simulink model "Nexonar_Navigation1"  (R2018b)
settings: Solver=FixedStepDiscrete  StartTime=0.0  StopTime=0.1  RelTol=1e-3  EnableMultiTasking=on
libraries: commutil2 x12, c280xlib x3, c2833xlib x2, c2000lib x1
settings Model: ExtModeTrigDuration=8  Creator=User  LastModifiedBy=hengw
settings DataIOCC: LimitDataPoints=on  SaveFormat=Array  SaveOutput=off  SaveTime=off
settings OptimizationCC: DefaultUnderspecifiedDataType=single  ExpressionDepthLimit=2147483647  LifeSpan=1  MaxStackSize=512
settings DebuggingCC: UnderspecifiedInitializationDetection=Classic  MergeDetectMultiDrivingBlocksExec=none  SolverPrmCheckMsg=warning  StateNameClashWarn=warning  SFUnexpectedBacktrackingDiag=warning  SFNoUnconditionalDefaultTransitionDiag=warning  SFExecutionAtInitializationDiag=none
settings HardwareCC: ProdBitPerChar=16  ProdBitPerInt=16  ProdBitPerPointer=32  ProdBitPerSizeT=32  ProdBitPerPtrDiffT=32  ProdLargestAtomicInteger=Integer  ProdLargestAtomicFloat=None  ProdWordSize=16  ProdLongLongMode=on  ProdHWDeviceType=Texas Instruments->C2000  TargetBitPerChar=16  TargetBitPerInt=16  TargetLargestAtomicInteger=Integer  TargetIntDivRoundTo=Zero  TargetEndianess=LittleEndian  TargetWordSize=16  TargetHWDeviceType=Texas Instruments->C2000  ProdEqTarget=off
settings ModelReferenceCC: PropagateSignalLabelsOutOfModel=off
settings SFSimCC: SimCustomSourceCode="#include \"i2c_reset.c\""  SimCustomHeaderCode="#include \"i2c_reset.h\""  SimUseLocalCustomCode=off  MATLABDynamicMemAlloc=off
settings RTWCC: SystemTargetFile=ert.tlc  HardwareBoard=TI Delfino F2833x  TemplateMakefile=ert_default_tmf  RTWUseLocalCustomCode=off  RTWUseSimCustomCode=on  CustomSourceCode="#include \"i2c_reset.c\""  CustomHeaderCode="#include \"i2c_reset.h\""  Toolchain=Texas Instruments Code Composer Studio (C2000)
settings CodeAppCC: IgnoreCustomStorageClasses=off  CustomSymbolStrType=$N$R$M  StateflowObjectComments=on  InternalIdentifier=Classic
settings ERTTargetCC: CodeReplacementLibrary=TI C28x  MultiwordLength=2048  ParMdlRefBuildCompliant=off  CPPClassGenCompliant=off  ConvertIfToSwitch=off  SuppressUnreachableDefaultCases=off
settings ConfigComp: CovMetricSettings=dw  CovHtmlReporting=on  CovSaveCumulativeToWorkspaceVar=on  CovSaveSingleToWorkspaceVar=on  CovExternalEMLEnable=off  PSAutoStubLUT=on

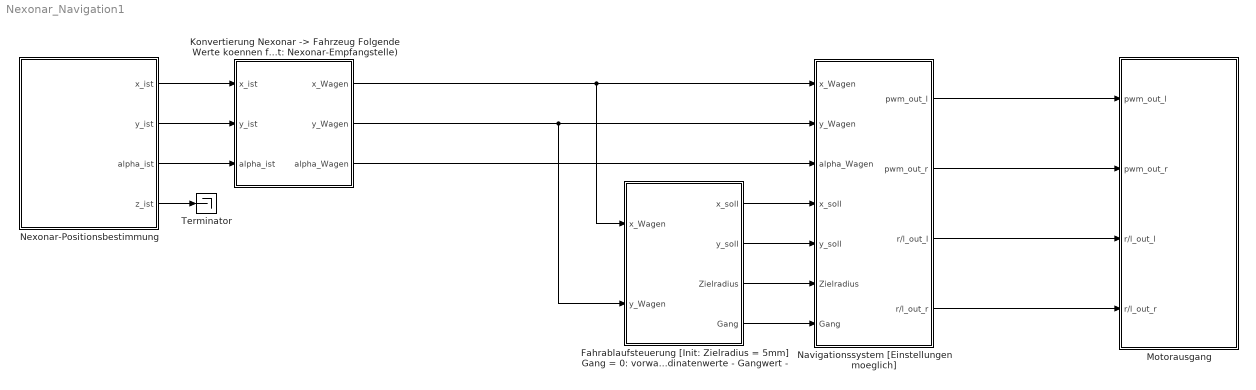
== system Nexonar_Navigation1 ==
  "Fahrablaufsteuerung [Init: Zielradius = 5mm] Gang = 0: vorwaerts Gang = 1: rueckwaerts Folgende Werte fuer den Ablauf sind einstellbar: - Zielkoordinatenwerte - Gangwert - " : Stateflow chart  TreatAsAtomicUnit=on
  "Konvertierung Nexonar -> Fahrzeug Folgende Werte koennen für Nexonar eingestellt werden: - r_Versatz_Nexo: Radialer Versatz des Nexonars zur Rotationsachse des Fahrzeugs - phi_Versatz_Nexo: Winkelversatz des Nexonars gegenüber der x-Achse (Mittelpunkt: Rotationspunkt des Fahrzeugs) - psi_Offset_Nexo: Winkelversatz des Nexonars gegenüber der x-Achse (Mittelpunkt: Nexonar-Empfangstelle)" : MATLAB Function  TreatAsAtomicUnit=on
  Motorausgang : Subsystem
  Navigationssystem [Einstellungen moeglich] : Subsystem  TreatAsAtomicUnit=on
  Nexonar-Positionsbestimmung : Subsystem
  Terminator : Terminator
  wires:
  Navigationssystem [Einstellungen moeglich]/2(pwm_out_r) -> Motorausgang/2(pwm_out_r)
  "Fahrablaufsteuerung [Init: Zielradius = 5mm] Gang = 0: vorwaerts Gang = 1: rueckwaerts Folgende Werte fuer den Ablauf sind einstellbar: - Zielkoordinatenwerte - Gangwert - "/2(y_soll) -> Navigationssystem [Einstellungen moeglich]/5(y_soll)
  Navigationssystem [Einstellungen moeglich]/3(r/l_out_l) -> Motorausgang/3(r/l_out_l)
  "Fahrablaufsteuerung [Init: Zielradius = 5mm] Gang = 0: vorwaerts Gang = 1: rueckwaerts Folgende Werte fuer den Ablauf sind einstellbar: - Zielkoordinatenwerte - Gangwert - "/4(Gang) -> Navigationssystem [Einstellungen moeglich]/7(Gang)
  "Fahrablaufsteuerung [Init: Zielradius = 5mm] Gang = 0: vorwaerts Gang = 1: rueckwaerts Folgende Werte fuer den Ablauf sind einstellbar: - Zielkoordinatenwerte - Gangwert - "/1(x_soll) -> Navigationssystem [Einstellungen moeglich]/4(x_soll)
  "Fahrablaufsteuerung [Init: Zielradius = 5mm] Gang = 0: vorwaerts Gang = 1: rueckwaerts Folgende Werte fuer den Ablauf sind einstellbar: - Zielkoordinatenwerte - Gangwert - "/3(Zielradius) -> Navigationssystem [Einstellungen moeglich]/6(Zielradius)
  "Konvertierung Nexonar -> Fahrzeug Folgende Werte koennen für Nexonar eingestellt werden: - r_Versatz_Nexo: Radialer Versatz des Nexonars zur Rotationsachse des Fahrzeugs - phi_Versatz_Nexo: Winkelversatz des Nexonars gegenüber der x-Achse (Mittelpunkt: Rotationspunkt des Fahrzeugs) - psi_Offset_Nexo: Winkelversatz des Nexonars gegenüber der x-Achse (Mittelpunkt: Nexonar-Empfangstelle)"/2(y_Wagen) -> "Fahrablaufsteuerung [Init: Zielradius = 5mm] Gang = 0: vorwaerts Gang = 1: rueckwaerts Folgende Werte fuer den Ablauf sind einstellbar: - Zielkoordinatenwerte - Gangwert - "/2(y_Wagen), Navigationssystem [Einstellungen moeglich]/2(y_Wagen)
  Navigationssystem [Einstellungen moeglich]/4(r/l_out_r) -> Motorausgang/4(r/l_out_r)
  "Konvertierung Nexonar -> Fahrzeug Folgende Werte koennen für Nexonar eingestellt werden: - r_Versatz_Nexo: Radialer Versatz des Nexonars zur Rotationsachse des Fahrzeugs - phi_Versatz_Nexo: Winkelversatz des Nexonars gegenüber der x-Achse (Mittelpunkt: Rotationspunkt des Fahrzeugs) - psi_Offset_Nexo: Winkelversatz des Nexonars gegenüber der x-Achse (Mittelpunkt: Nexonar-Empfangstelle)"/1(x_Wagen) -> "Fahrablaufsteuerung [Init: Zielradius = 5mm] Gang = 0: vorwaerts Gang = 1: rueckwaerts Folgende Werte fuer den Ablauf sind einstellbar: - Zielkoordinatenwerte - Gangwert - "/1(x_Wagen), Navigationssystem [Einstellungen moeglich]/1(x_Wagen)
  Navigationssystem [Einstellungen moeglich]/1(pwm_out_l) -> Motorausgang/1(pwm_out_l)
  Nexonar-Positionsbestimmung/4(z_ist) -> Terminator/1
  "Konvertierung Nexonar -> Fahrzeug Folgende Werte koennen für Nexonar eingestellt werden: - r_Versatz_Nexo: Radialer Versatz des Nexonars zur Rotationsachse des Fahrzeugs - phi_Versatz_Nexo: Winkelversatz des Nexonars gegenüber der x-Achse (Mittelpunkt: Rotationspunkt des Fahrzeugs) - psi_Offset_Nexo: Winkelversatz des Nexonars gegenüber der x-Achse (Mittelpunkt: Nexonar-Empfangstelle)"/3(alpha_Wagen) -> Navigationssystem [Einstellungen moeglich]/3(alpha_Wagen)
  Nexonar-Positionsbestimmung/1(x_ist) -> "Konvertierung Nexonar -> Fahrzeug Folgende Werte koennen für Nexonar eingestellt werden: - r_Versatz_Nexo: Radialer Versatz des Nexonars zur Rotationsachse des Fahrzeugs - phi_Versatz_Nexo: Winkelversatz des Nexonars gegenüber der x-Achse (Mittelpunkt: Rotationspunkt des Fahrzeugs) - psi_Offset_Nexo: Winkelversatz des Nexonars gegenüber der x-Achse (Mittelpunkt: Nexonar-Empfangstelle)"/1(x_ist)
  Nexonar-Positionsbestimmung/2(y_ist) -> "Konvertierung Nexonar -> Fahrzeug Folgende Werte koennen für Nexonar eingestellt werden: - r_Versatz_Nexo: Radialer Versatz des Nexonars zur Rotationsachse des Fahrzeugs - phi_Versatz_Nexo: Winkelversatz des Nexonars gegenüber der x-Achse (Mittelpunkt: Rotationspunkt des Fahrzeugs) - psi_Offset_Nexo: Winkelversatz des Nexonars gegenüber der x-Achse (Mittelpunkt: Nexonar-Empfangstelle)"/2(y_ist)
  Nexonar-Positionsbestimmung/3(alpha_ist) -> "Konvertierung Nexonar -> Fahrzeug Folgende Werte koennen für Nexonar eingestellt werden: - r_Versatz_Nexo: Radialer Versatz des Nexonars zur Rotationsachse des Fahrzeugs - phi_Versatz_Nexo: Winkelversatz des Nexonars gegenüber der x-Achse (Mittelpunkt: Rotationspunkt des Fahrzeugs) - psi_Offset_Nexo: Winkelversatz des Nexonars gegenüber der x-Achse (Mittelpunkt: Nexonar-Empfangstelle)"/3(alpha_ist)

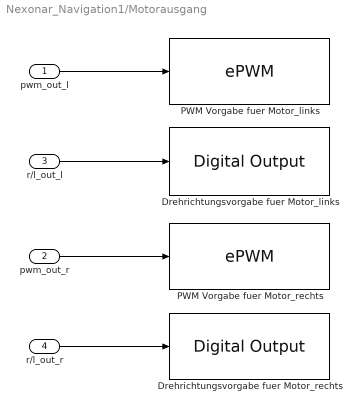
== system Nexonar_Navigation1/Motorausgang ==
  pwm_out_l : Inport
  pwm_out_r : Inport  Port=2
  r/l_out_l : Inport  Port=3
  r/l_out_r : Inport  Port=4
  Drehrichtungsvorgabe fuer Motor_links : c2833xlib/Digital Output  GPIO_Number=GPIO16~GPIO23  GPIO_Bit0=off  GPIO_BIT0_Toggle=off  GPIO_Bit1=off  GPIO_BIT1_Toggle=off  GPIO_Bit2=off  GPIO_BIT2_Toggle=off  GPIO_Bit3=off  GPIO_BIT3_Toggle=off  GPIO_Bit4=on  GPIO_BIT4_Toggle=off  GPIO_Bit5=off  GPIO_BIT5_Toggle=off  GPIO_Bit6=off  GPIO_BIT6_Toggle=off  GPIO_Bit7=off  GPIO_BIT7_Toggle=off
      settings: SourceProductName=Embedded Coder Support Package for Texas Instruments C2000 Processors  SourceProductBaseCode=TIC2000
  Drehrichtungsvorgabe fuer Motor_rechts : c2833xlib/Digital Output  GPIO_Number=GPIO16~GPIO23  GPIO_Bit0=off  GPIO_BIT0_Toggle=off  GPIO_Bit1=off  GPIO_BIT1_Toggle=off  GPIO_Bit2=off  GPIO_BIT2_Toggle=off  GPIO_Bit3=off  GPIO_BIT3_Toggle=off  GPIO_Bit4=off  GPIO_BIT4_Toggle=off  GPIO_Bit5=on  GPIO_BIT5_Toggle=off  GPIO_Bit6=off  GPIO_BIT6_Toggle=off  GPIO_Bit7=off  GPIO_BIT7_Toggle=off
      settings: SourceProductName=Embedded Coder Support Package for Texas Instruments C2000 Processors  SourceProductBaseCode=TIC2000
  "PWM Vorgabe fuer Motor_links " : c280xlib/ePWM  checkMode=off  useModule=ePWM1  periodUnits=Clock cycles  timerSource=Specify via dialog  timerPeriod_clk=64000  timerPeriod_sec=0.0001  tbshadow=Counter equals to zero  countingMode=Up  phaseActiveEnable=Disable  phaseDirection=Count down after sync  phaseActive=0  synchronizationEnable=off  synchronizationOption=Disable  clockPrescale=1  HSclockPrescale=1  ePWMxAStatus=off  CMPAUnits=Clock cycles  CMPASource=Specify via dialog  CMPAValue_per=50  CMPAValue_clk=32000  enCMPAshadow=Counter equals to zero  ePWMxAactionLogic1=Do nothing  ePWMxAactionLogic2=Clear  ePWMxAactionLogic3=Set  ePWMxAactionLogic4=Do nothing  ePWMxAactionLogic5=Do nothing  ePWMxAactionLogic6=Do nothing  ePWMxALoadMode=Load on counter equals to zero (CTR=Zero)  ePWMxACSFenable=off  ePWMxACSFvalue=Forcing disable  ePWMxASFreload=Zero  enHRPWM=off  HRPWM_LoadMode=Counter equals to zero (CTR=ZERO)  HRPWM_CTLMode=Phase control mode  HRPWM_EDGMode=Both edge  enSFO=on  ePWMxBStatus=on  CMPBUnits=Percentages  CMPBSource=Input port  CMPBValue_per=0  CMPBValue_clk=32000  enCMPBshadow=Counter equals to zero  ePWMxBactionLogic1=Do nothing  ePWMxBactionLogic2=Set  ePWMxBactionLogic3=Do nothing  ePWMxBactionLogic4=Do nothing  ePWMxBactionLogic5=Clear  ePWMxBactionLogic6=Do nothing  ePWMxBLoadMode=Load on counter equals to zero (CTR=Zero)  ePWMxBCSFenable=off  ePWMxBCSFvalue=Forcing disable  ePWMxBSFreload=Zero  enableDBePWMxA=off  enableDBePWMxB=off  DBpolarity=Active high (AH)  DBedgeDelay=Positive  DBSource_ePWMxA=ePWMxA  DBSource_ePWMxB=ePWMxA  DBperiodSource=Specify via dialog  REDperiod=0  FEDperiod=0  adcstartModuleA=off  adcrequestEventA=First event  adcstartEventA=Counter equals to zero (CTR=Zero)  adcstartModuleB=off  adcrequestEventB=First event  adcstartEventB=Counter equals to zero (CTR=Zero)  intEn=off  intPrd=First event  intSel=Counter equals to zero (CTR=Zero)  chopperEnable=off  chopperFrequency=1  chopperFirstwidth=1  chopperDuty=12.5%  tripZonesource=Specify via dialog  tzselOSHT1=off  tzselOSHT2=off  tzselOSHT3=off  tzselOSHT4=off  tzselOSHT5=off  tzselOSHT6=off  tzselCBC1=off  tzselCBC2=off  tzselCBC3=off  tzselCBC4=off  tzselCBC5=off  tzselCBC6=off  enTzOstIntr=off  enTzCbcIntr=off  ePWMxAforced=No action  ePWMxBforced=No action  timerPeriod=-1  ePWMxAValue=0  ePWMxBValue=0  tripZoneoption=One-shot trip (OSHT)
      settings: SourceProductName=Embedded Coder Support Package for Texas Instruments C2000 Processors  SourceProductBaseCode=TIC2000
  PWM Vorgabe fuer Motor_rechts : c280xlib/ePWM  checkMode=off  useModule=ePWM2  periodUnits=Clock cycles  timerSource=Specify via dialog  timerPeriod_clk=64000  timerPeriod_sec=0.0001  tbshadow=Counter equals to zero  countingMode=Up  phaseActiveEnable=Disable  phaseDirection=Count down after sync  phaseActive=0  synchronizationEnable=off  synchronizationOption=Disable  clockPrescale=1  HSclockPrescale=1  ePWMxAStatus=off  CMPAUnits=Clock cycles  CMPASource=Specify via dialog  CMPAValue_per=50  CMPAValue_clk=32000  enCMPAshadow=Counter equals to zero  ePWMxAactionLogic1=Do nothing  ePWMxAactionLogic2=Clear  ePWMxAactionLogic3=Set  ePWMxAactionLogic4=Do nothing  ePWMxAactionLogic5=Do nothing  ePWMxAactionLogic6=Do nothing  ePWMxALoadMode=Load on counter equals to zero (CTR=Zero)  ePWMxACSFenable=off  ePWMxACSFvalue=Forcing disable  ePWMxASFreload=Zero  enHRPWM=off  HRPWM_LoadMode=Counter equals to zero (CTR=ZERO)  HRPWM_CTLMode=Phase control mode  HRPWM_EDGMode=Both edge  enSFO=on  ePWMxBStatus=on  CMPBUnits=Percentages  CMPBSource=Input port  CMPBValue_per=0  CMPBValue_clk=32000  enCMPBshadow=Counter equals to zero  ePWMxBactionLogic1=Do nothing  ePWMxBactionLogic2=Set  ePWMxBactionLogic3=Do nothing  ePWMxBactionLogic4=Do nothing  ePWMxBactionLogic5=Clear  ePWMxBactionLogic6=Do nothing  ePWMxBLoadMode=Load on counter equals to zero (CTR=Zero)  ePWMxBCSFenable=off  ePWMxBCSFvalue=Forcing disable  ePWMxBSFreload=Zero  enableDBePWMxA=off  enableDBePWMxB=off  DBpolarity=Active high (AH)  DBedgeDelay=Positive  DBSource_ePWMxA=ePWMxA  DBSource_ePWMxB=ePWMxA  DBperiodSource=Specify via dialog  REDperiod=0  FEDperiod=0  adcstartModuleA=off  adcrequestEventA=First event  adcstartEventA=Counter equals to zero (CTR=Zero)  adcstartModuleB=off  adcrequestEventB=First event  adcstartEventB=Counter equals to zero (CTR=Zero)  intEn=off  intPrd=First event  intSel=Counter equals to zero (CTR=Zero)  chopperEnable=off  chopperFrequency=1  chopperFirstwidth=1  chopperDuty=12.5%  tripZonesource=Specify via dialog  tzselOSHT1=off  tzselOSHT2=off  tzselOSHT3=off  tzselOSHT4=off  tzselOSHT5=off  tzselOSHT6=off  tzselCBC1=off  tzselCBC2=off  tzselCBC3=off  tzselCBC4=off  tzselCBC5=off  tzselCBC6=off  enTzOstIntr=off  enTzCbcIntr=off  ePWMxAforced=No action  ePWMxBforced=No action  timerPeriod=-1  ePWMxAValue=0  ePWMxBValue=0  tripZoneoption=One-shot trip (OSHT)
      settings: SourceProductName=Embedded Coder Support Package for Texas Instruments C2000 Processors  SourceProductBaseCode=TIC2000
  wires:
  pwm_out_l/1 -> "PWM Vorgabe fuer Motor_links "/1
  pwm_out_r/1 -> PWM Vorgabe fuer Motor_rechts/1
  r/l_out_l/1 -> Drehrichtungsvorgabe fuer Motor_links/1
  r/l_out_r/1 -> Drehrichtungsvorgabe fuer Motor_rechts/1

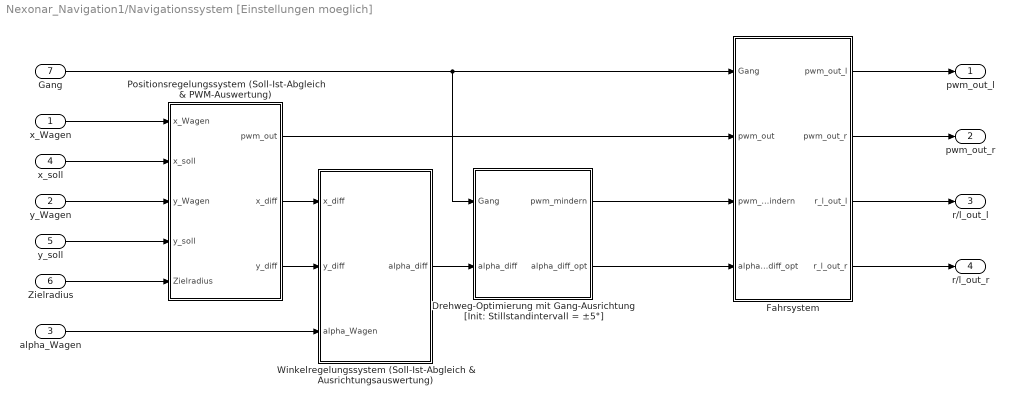
== system Nexonar_Navigation1/Navigationssystem [Einstellungen moeglich] ==
  x_Wagen : Inport
  y_Wagen : Inport  Port=2
  alpha_Wagen : Inport  Port=3
  x_soll : Inport  Port=4
  y_soll : Inport  Port=5
  Zielradius : Inport  Port=6
  Gang : Inport  Port=7
  Drehweg-Optimierung mit Gang-Ausrichtung [Init: Stillstandintervall = ±5°] : Stateflow chart  TreatAsAtomicUnit=on
  Fahrsystem : Stateflow chart  TreatAsAtomicUnit=on
  Positionsregelungssystem (Soll-Ist-Abgleich & PWM-Auswertung) : Subsystem
  Winkelregelungssystem (Soll-Ist-Abgleich & Ausrichtungsauswertung) : Subsystem
  pwm_out_l : Outport
  pwm_out_r : Outport  Port=2
  r/l_out_l : Outport  Port=3
  r/l_out_r : Outport  Port=4
  wires:
  Positionsregelungssystem (Soll-Ist-Abgleich & PWM-Auswertung)/2(x_diff) -> Winkelregelungssystem (Soll-Ist-Abgleich & Ausrichtungsauswertung)/1(x_diff)
  y_soll/1 -> Positionsregelungssystem (Soll-Ist-Abgleich & PWM-Auswertung)/4(y_soll)
  y_Wagen/1 -> Positionsregelungssystem (Soll-Ist-Abgleich & PWM-Auswertung)/3(y_Wagen)
  Gang/1 -> Fahrsystem/1(Gang), Drehweg-Optimierung mit Gang-Ausrichtung [Init: Stillstandintervall = ±5°]/1(Gang)
  Positionsregelungssystem (Soll-Ist-Abgleich & PWM-Auswertung)/3(y_diff) -> Winkelregelungssystem (Soll-Ist-Abgleich & Ausrichtungsauswertung)/2(y_diff)
  x_Wagen/1 -> Positionsregelungssystem (Soll-Ist-Abgleich & PWM-Auswertung)/1(x_Wagen)
  x_soll/1 -> Positionsregelungssystem (Soll-Ist-Abgleich & PWM-Auswertung)/2(x_soll)
  alpha_Wagen/1 -> Winkelregelungssystem (Soll-Ist-Abgleich & Ausrichtungsauswertung)/3(alpha_Wagen)
  Fahrsystem/2(pwm_out_r) -> pwm_out_r/1
  Fahrsystem/4(r_l_out_r) -> r/l_out_r/1
  Fahrsystem/1(pwm_out_l) -> pwm_out_l/1
  Fahrsystem/3(r_l_out_l) -> r/l_out_l/1
  Winkelregelungssystem (Soll-Ist-Abgleich & Ausrichtungsauswertung)/1(alpha_diff) -> Drehweg-Optimierung mit Gang-Ausrichtung [Init: Stillstandintervall = ±5°]/2(alpha_diff)
  Drehweg-Optimierung mit Gang-Ausrichtung [Init: Stillstandintervall = ±5°]/2(alpha_diff_opt) -> Fahrsystem/4(alpha_diff_opt)
  Zielradius/1 -> Positionsregelungssystem (Soll-Ist-Abgleich & PWM-Auswertung)/5(Zielradius)
  Drehweg-Optimierung mit Gang-Ausrichtung [Init: Stillstandintervall = ±5°]/1(pwm_mindern) -> Fahrsystem/3(pwm_mindern)
  Positionsregelungssystem (Soll-Ist-Abgleich & PWM-Auswertung)/1(pwm_out) -> Fahrsystem/2(pwm_out)

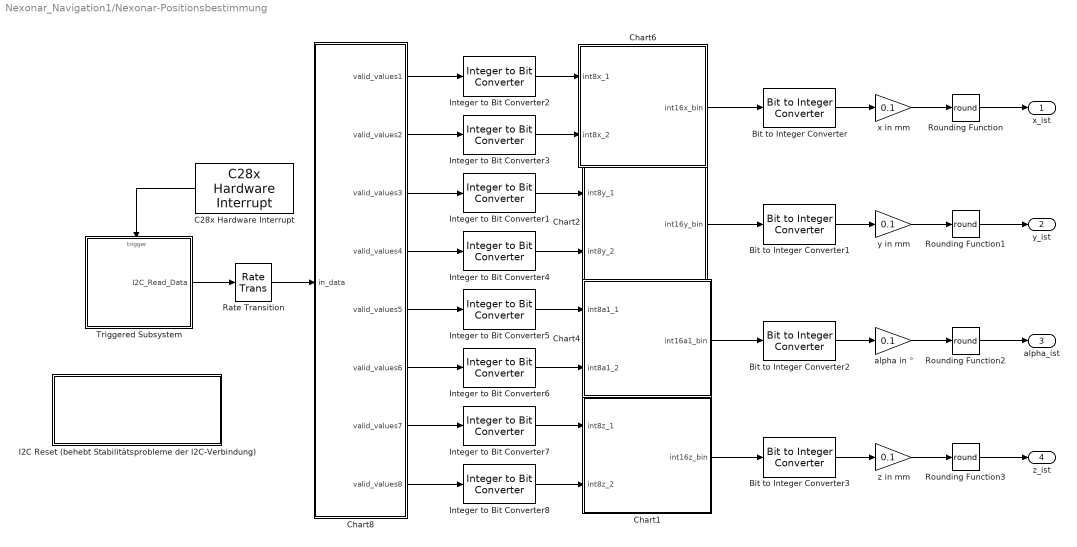
== system Nexonar_Navigation1/Nexonar-Positionsbestimmung ==
  Bit to Integer Converter{,1..3} (4 alike) : commutil2/Bit to Integer Converter  nbits=16  bitOrder=MSB first  signedOutputValues=Signed  outDtype=Inherit via internal rule  outDtypeSigned=Inherit via internal rule
      settings: SourceProductName=Communications Toolbox
  C28x Hardware Interrupt : c2000lib/Scheduling/C28x Hardware Interrupt  irqnumbers=8  pienumbers=2  irqpriorities=30  irqpreempts=0  showinput=off  dspchiptype=C280X
      settings: SourceProductName=Embedded Coder Support Package for Texas Instruments C2000 Processors  SourceProductBaseCode=TIC2000
  Chart1 : Stateflow chart  TreatAsAtomicUnit=on
  Chart2 : Stateflow chart  TreatAsAtomicUnit=on
  Chart4 : Stateflow chart  TreatAsAtomicUnit=on
  Chart6 : Stateflow chart  TreatAsAtomicUnit=on
  Chart8 : Stateflow chart  TreatAsAtomicUnit=on
  I2C Reset (behebt Stabilitätsprobleme der I2C-Verbindung) : Subsystem
  Integer to Bit Converter{1..8} (8 alike) : commutil2/Integer to Bit Converter  nbits=8  signedInputValues=Unsigned  bitOrder=MSB first  outDtype=uint8
      settings: SourceProductName=Communications Toolbox
  Rate Transition : RateTransition  Deterministic=off  OutPortSampleTime=0.01
  Rounding Function{,1..3} (4 alike) : Rounding  Operator=round
  Triggered Subsystem : Subsystem  TreatAsAtomicUnit=on
  alpha in ° : Gain  Gain=0.1  OutDataTypeStr=double
  x in mm : Gain  Gain=0.1  OutDataTypeStr=double
  y in mm : Gain  Gain=0.1  OutDataTypeStr=double
  z in mm : Gain  Gain=0.1  OutDataTypeStr=double
  x_ist : Outport
  y_ist : Outport  Port=2
  alpha_ist : Outport  Port=3
  z_ist : Outport  Port=4
  wires:
  Integer to Bit Converter7/1 -> Chart1/1(int8z_1)
  Integer to Bit Converter8/1 -> Chart1/2(int8z_2)
  Chart8/7(valid_values7) -> Integer to Bit Converter7/1
  Chart8/8(valid_values8) -> Integer to Bit Converter8/1
  Triggered Subsystem/1(I2C_Read_Data) -> Rate Transition/1
  Chart1/1(int16z_bin) -> Bit to Integer Converter3/1
  Chart4/1(int16a1_bin) -> Bit to Integer Converter2/1
  Chart8/6(valid_values6) -> Integer to Bit Converter6/1
  Integer to Bit Converter6/1 -> Chart4/2(int8a1_2)
  Integer to Bit Converter5/1 -> Chart4/1(int8a1_1)
  Integer to Bit Converter4/1 -> Chart2/2(int8y_2)
  Integer to Bit Converter2/1 -> Chart6/1(int8x_1)
  Integer to Bit Converter1/1 -> Chart2/1(int8y_1)
  Chart6/1(int16x_bin) -> Bit to Integer Converter/1
  Integer to Bit Converter3/1 -> Chart6/2(int8x_2)
  Chart8/3(valid_values3) -> Integer to Bit Converter1/1
  Chart8/1(valid_values1) -> Integer to Bit Converter2/1
  Chart2/1(int16y_bin) -> Bit to Integer Converter1/1
  Chart8/4(valid_values4) -> Integer to Bit Converter4/1
  Chart8/2(valid_values2) -> Integer to Bit Converter3/1
  Chart8/5(valid_values5) -> Integer to Bit Converter5/1
  C28x Hardware Interrupt/1 -> Triggered Subsystem/Trigger
  Rate Transition/1 -> Chart8/1(in_data)
  x in mm/1 -> Rounding Function/1
  Bit to Integer Converter/1 -> x in mm/1
  Bit to Integer Converter1/1 -> y in mm/1
  y in mm/1 -> Rounding Function1/1
  Bit to Integer Converter3/1 -> z in mm/1
  z in mm/1 -> Rounding Function3/1
  Bit to Integer Converter2/1 -> alpha in °/1
  alpha in °/1 -> Rounding Function2/1
  Rounding Function/1 -> x_ist/1
  Rounding Function2/1 -> alpha_ist/1
  Rounding Function1/1 -> y_ist/1
  Rounding Function3/1 -> z_ist/1

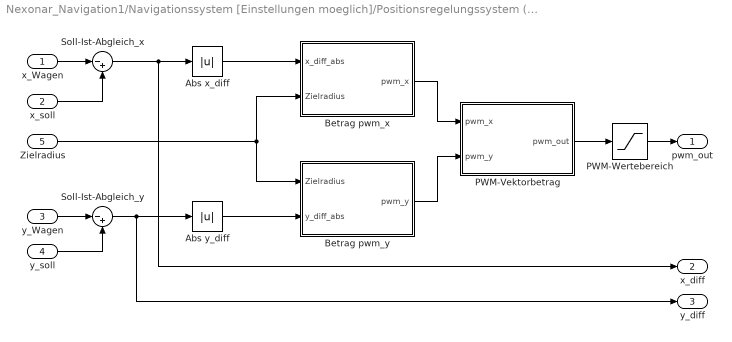
== system Nexonar_Navigation1/Navigationssystem [Einstellungen moeglich]/Positionsregelungssystem (Soll-Ist-Abgleich & PWM-Auswertung) ==
  x_Wagen : Inport
  x_soll : Inport  Port=2
  y_Wagen : Inport  Port=3
  y_soll : Inport  Port=4
  Zielradius : Inport  Port=5
  Abs x_diff : Abs  SampleTime=0.01
  Abs y_diff : Abs  SampleTime=0.01
  Betrag pwm_x : MATLAB Function  TreatAsAtomicUnit=on  SystemSampleTime=0.01
  Betrag pwm_y : MATLAB Function  TreatAsAtomicUnit=on  SystemSampleTime=0.01
  PWM-Vektorbetrag : MATLAB Function  TreatAsAtomicUnit=on
  PWM-Wertebereich : Saturate  UpperLimit=100  LowerLimit=0
  Soll-Ist-Abgleich_x : Sum  Inputs=|-+  SampleTime=0.01
  Soll-Ist-Abgleich_y : Sum  Inputs=|-+  AccumDataTypeStr=double  SampleTime=0.01
  pwm_out : Outport
  x_diff : Outport  Port=2
  y_diff : Outport  Port=3
  wires:
  Soll-Ist-Abgleich_x/1 -> x_diff/1, Abs x_diff/1
  Abs x_diff/1 -> Betrag pwm_x/1(x_diff_abs)
  x_soll/1 -> Soll-Ist-Abgleich_x/2
  x_Wagen/1 -> Soll-Ist-Abgleich_x/1
  y_Wagen/1 -> Soll-Ist-Abgleich_y/1
  y_soll/1 -> Soll-Ist-Abgleich_y/2
  Soll-Ist-Abgleich_y/1 -> Abs y_diff/1, y_diff/1
  Abs y_diff/1 -> Betrag pwm_y/2(y_diff_abs)
  PWM-Wertebereich/1 -> pwm_out/1
  PWM-Vektorbetrag/1(pwm_out) -> PWM-Wertebereich/1
  Betrag pwm_x/1(pwm_x) -> PWM-Vektorbetrag/1(pwm_x)
  Betrag pwm_y/1(pwm_y) -> PWM-Vektorbetrag/2(pwm_y)
  Zielradius/1 -> Betrag pwm_y/1(Zielradius), Betrag pwm_x/2(Zielradius)

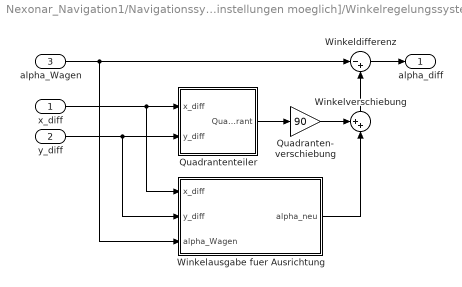
== system Nexonar_Navigation1/Navigationssystem [Einstellungen moeglich]/Winkelregelungssystem (Soll-Ist-Abgleich & Ausrichtungsauswertung) ==
  x_diff : Inport
  y_diff : Inport  Port=2
  alpha_Wagen : Inport  Port=3
  Quadranten- verschiebung : Gain  Gain=90
  Quadrantenteiler : Stateflow chart  TreatAsAtomicUnit=on
  Winkelausgabe fuer Ausrichtung : Stateflow chart  TreatAsAtomicUnit=on
  Winkeldifferenz : Sum  Inputs=|-+
  Winkelverschiebung : Sum  Inputs=++|
  alpha_diff : Outport
  wires:
  alpha_Wagen/1 -> Winkelausgabe fuer Ausrichtung/3(alpha_Wagen), Winkeldifferenz/1
  y_diff/1 -> Winkelausgabe fuer Ausrichtung/2(y_diff), Quadrantenteiler/2(y_diff)
  Winkelausgabe fuer Ausrichtung/1(alpha_neu) -> Winkelverschiebung/2
  Winkelverschiebung/1 -> Winkeldifferenz/2
  x_diff/1 -> Winkelausgabe fuer Ausrichtung/1(x_diff), Quadrantenteiler/1(x_diff)
  Quadrantenteiler/1(Quadrant) -> Quadranten- verschiebung/1
  Winkeldifferenz/1 -> alpha_diff/1
  Quadranten- verschiebung/1 -> Winkelverschiebung/1

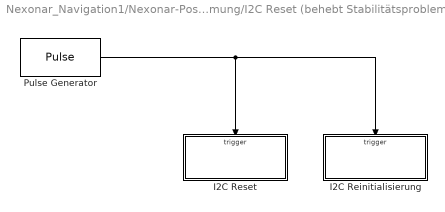
== system Nexonar_Navigation1/Nexonar-Positionsbestimmung/I2C Reset (behebt Stabilitätsprobleme der I2C-Verbindung) ==
  I2C Reinitialisierung : Subsystem  TreatAsAtomicUnit=on
  I2C Reset : Subsystem  TreatAsAtomicUnit=on
  Pulse Generator : DiscretePulseGenerator  Period=250  SampleTime=0.01
  wires:
  Pulse Generator/1 -> I2C Reinitialisierung/Trigger, I2C Reset/Trigger

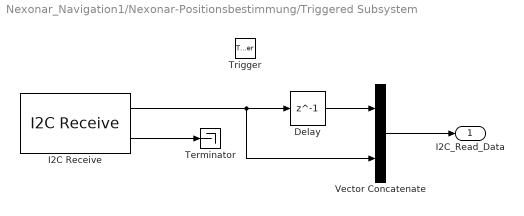
== system Nexonar_Navigation1/Nexonar-Positionsbestimmung/Triggered Subsystem ==
  Trigger : TriggerPort  TriggerType=function-call  VariantControl=(inherit)
  Delay : Delay  DelayLength=1  InitialCondition=0
  I2C Receive : c280xlib/I2C Receive  selectModule=I2C_A  addrFormat=7-Bit addressing  saSource=Specify via dialog  SAR=80  bitCount=8  dataLength=10  initValue=0  NACK=on  STP=off  STR=on  sampleTime=-1  dataType=uint8
      settings: SourceProductName=Embedded Coder Support Package for Texas Instruments C2000 Processors  SourceProductBaseCode=TIC2000
  Terminator : Terminator
  Vector Concatenate : Concatenate
  I2C_Read_Data : Outport
  wires:
  I2C Receive/2 -> Terminator/1
  I2C Receive/1 -> Vector Concatenate/2, Delay/1
  Delay/1 -> Vector Concatenate/1
  Vector Concatenate/1 -> I2C_Read_Data/1

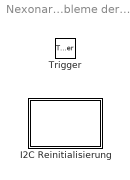
== system Nexonar_Navigation1/Nexonar-Positionsbestimmung/I2C Reset (behebt Stabilitätsprobleme der I2C-Verbindung)/I2C Reinitialisierung ==
  Trigger : TriggerPort  TriggerType=falling  VariantControl=(inherit)
  I2C Reinitialisierung : MATLAB Function  TreatAsAtomicUnit=on

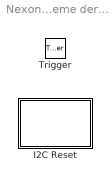
== system Nexonar_Navigation1/Nexonar-Positionsbestimmung/I2C Reset (behebt Stabilitätsprobleme der I2C-Verbindung)/I2C Reset ==
  Trigger : TriggerPort  VariantControl=(inherit)
  I2C Reset : MATLAB Function  TreatAsAtomicUnit=on

== stateflow chart Nexonar_Navigation1/Nexonar-Positionsbestimmung/Chart1 ==
  state Daten_einlesen
  state x0
  state x1_1
    entry: int16z_bin[0] = int8z_1[0];
    int16z_bin[1] = int8z_1[1];
    int16z_bin[2] = int8z_1[2];
    int16z_bin[3] = int8z_1[3];
    int16z_bin[4] = int8z_1[4];
    int16z_bin[5] = int8z_1[5]
    int16z_bin[6] = int8z_1[6];
    int16z_bin[7] = int8z_1[7];
    int16z_bin[8] = int8z_2[0];
    int16z_bin[9] = int8z_2[1];
    int16z_bin[10] = int8z_2[2];
    int16z_bin[11] = int8z_2[3];
    int16z_bin[12] = int8z_2[4];
    int16z_bin[13] = int8z_2[5]
    int16z_bin[14] = int8z_2[6];
    int16z_bin[15] = int8z_2[7];
  x0 -> Daten_einlesen
  (default) -> x0
  Daten_einlesen -> x1_1
  x1_1 -> Daten_einlesen
  data: int8z_1 input size=8; int8z_2 input size=8; int16z_bin output size=16 =0

== matlab function Nexonar_Navigation1/Navigationssystem [Einstellungen moeglich]/Positionsregelungssystem (Soll-Ist-Abgleich & PWM-Auswertung)/PWM-Vektorbetrag ==
  data: pwm_x input; pwm_out output; pwm_y input
function pwm_out = fcn(pwm_x, pwm_y)

pwm_out = round(sqrt(pwm_x * pwm_x + pwm_y * pwm_y));

== matlab function Nexonar_Navigation1/Konvertierung Nexonar -> Fahrzeug Folgende Werte koennen für Nexonar eingestellt werden: - r_Versatz_Nexo: Radialer Versatz des Nexonars zur Rotationsachse des Fahrzeugs - phi_Versatz_Nexo: Winkelversatz des Nexonars gegenüber der x-Achse (Mittelpunkt: Rotationspunkt des Fahrzeugs) - psi_Offset_Nexo: Winkelversatz des Nexonars gegenüber der x-Achse (Mittelpunkt: Nexonar-Empfangstelle) ==
  data: x_ist input; x_Wagen output; y_ist input; alpha_ist input; y_Wagen output; alpha_Wagen output
function [x_Wagen, y_Wagen, alpha_Wagen] = fcn(x_ist, y_ist, alpha_ist)

r_Versatz_Nexo = 2.5; % in mm
phi_Versatz_Nexo = 30; % in °
psi_Offset_Nexo = 15; % in 


alpha_Wagen = alpha_ist - psi_Offset_Nexo;
x_Wagen = x_ist - round(r_Versatz_Nexo * cos((phi_Versatz_Nexo+alpha_Wagen)*2*pi/360));
y_Wagen = y_ist - round(r_Versatz_Nexo * sin((phi_Versatz_Nexo+alpha_Wagen)*2*pi/360));

== stateflow chart Nexonar_Navigation1/Fahrablaufsteuerung [Init: Zielradius = 5mm] Gang = 0: vorwaerts Gang = 1: rueckwaerts Folgende Werte fuer den Ablauf sind einstellbar: - Zielkoordinatenwerte - Gangwert -  ==
  state Parken
    state Parken_1
      entry:
      x_soll = 1440;
      y_soll = -50;
    state Wechsel_1
      entry:
      Counter = Counter + 1;
    state Parken_2
      entry:
      x_soll = 1640;
      y_soll = -150;
    state Wechsel_2
      entry:
      Counter = Counter + 1;
    state Parken_3
      entry:
      x_soll = 1660;
      y_soll = -140;
    state Wechsel_3
      entry:
      Counter = Counter + 1;
    (default) -> Parken_1 : {Counter = 0}
    Parken_1 -> Parken.Wechsel_1 : [abs(x_soll - x_Wagen) <= Zielradius && abs(y_soll - y_Wagen) <= Zielradius]
    Parken.Wechsel_1 -> Parken_2
    Parken_2 -> Parken.Wechsel_2 : [abs(x_soll - x_Wagen) <= Zielradius && abs(y_soll - y_Wagen) <= Zielradius]
    Parken.Wechsel_2 -> Parken_3
    Parken_3 -> Parken.Wechsel_3 : [abs(x_soll - x_Wagen) <= Zielradius && abs(y_soll - y_Wagen) <= Zielradius]
  state Uebergabe
    state Uebergabepunkt_x_Richtung
      entry:
      x_soll = 1320;
      y_soll = y_least;
    state Wechsel_1
      entry:
      Counter = Counter + 1;
    state Uebergabepunkt_y_Richtung
      entry:
      x_soll = x_least;
      y_soll = 100;
    state Warten_Uebergabe
    state Wechsel_2
      entry:
      Counter = Counter + 1;
    (default) -> Uebergabepunkt_x_Richtung : {Counter = 0}
    Uebergabepunkt_x_Richtung -> Uebergabe.Wechsel_1 : [abs(x_soll - x_Wagen) <= Zielradius && abs(y_soll - y_Wagen) <= Zielradius]
        | {x_least = x_soll; y_least = y_soll;}
    Uebergabe.Wechsel_1 -> Uebergabepunkt_y_Richtung
    Uebergabepunkt_y_Richtung -> Warten_Uebergabe : [abs(x_soll - x_Wagen) <= Zielradius && abs(y_soll - y_Wagen) <= Zielradius]
    Warten_Uebergabe -> Uebergabe.Wechsel_2 : [after(1,sec)]
  state Start_Einstellung_Init
    entry:
    Zielradius = 20;
  state Sammeln
    state Anfahrpunkt_1
      entry:
      x_soll = 1500;
      y_soll = 0;
    state Wechsel_1
      entry:
      Counter = Counter + 1;
    state Anfahrpunkt_2
      entry:
      x_soll = 1000;
      y_soll = 100;
    state Wechsel_2
      entry:
      Counter = Counter + 1;
    state Anfahrpunkt_3
      entry:
      x_soll = 950;
      y_soll = 650;
    state Wechsel_3
      entry:
      Counter = Counter + 1;
    state Anfahrpunkt_4
      entry:
      x_soll = 850;
      y_soll = 800;
    state Wechsel_4
      entry:
      Counter = Counter + 1;
    state Anfahrpunkt_5
      entry:
      x_soll = 600;
      y_soll = 825;
    state Wechsel_5
      entry:
      Counter = Counter + 1;
    state Anfahrpunkt_6
      entry:
      x_soll = 500;
      y_soll = 825;
    state Wechsel_6
      entry:
      Counter = Counter + 1;
    state Anfahrpunkt_7
      entry:
      x_soll = 325;
      y_soll = 750;
    state Wechsel_7
      entry:
      Counter = Counter + 1;
    state Anfahrpunkt_8
      entry:
      x_soll = 275;
      y_soll = 725;
    state Wechsel_8
      entry:
      Counter = Counter + 1;
    state Anfahrpunkt_9
      entry:
      x_soll = 400;
      y_soll = 50;
    state Wechsel_9
      entry:
      Counter = Counter + 1;
    state Anfahrpunkt_10
      entry:
      x_soll = 1200;
      y_soll = 50;
    state Wechsel_10
      entry:
      Counter = Counter + 1;
    state Anfahrpunkt_11
      entry:
      x_soll = 1340;
      y_soll = -50;
    state Wechsel_11
      entry:
      Counter = Counter + 1;
    (default) -> Anfahrpunkt_1 : {Counter = 0}
    Anfahrpunkt_1 -> Sammeln.Wechsel_1 : [abs(x_soll - x_Wagen) <= Zielradius && abs(y_soll - y_Wagen) <= Zielradius]
    Sammeln.Wechsel_1 -> Anfahrpunkt_2
    Anfahrpunkt_2 -> Sammeln.Wechsel_2 : [abs(x_soll - x_Wagen) <= Zielradius && abs(y_soll - y_Wagen) <= Zielradius]
    Sammeln.Wechsel_2 -> Anfahrpunkt_3
    Wechsel_9 -> Anfahrpunkt_3 [order 1] : [Counter == 9]
    Anfahrpunkt_3 -> Sammeln.Wechsel_3 : [abs(x_soll - x_Wagen) <= Zielradius && abs(y_soll - y_Wagen) <= Zielradius]
    Sammeln.Wechsel_3 -> Anfahrpunkt_4
    Anfahrpunkt_4 -> Wechsel_4 : [abs(x_soll - x_Wagen) <= Zielradius && abs(y_soll - y_Wagen) <= Zielradius]
    Wechsel_4 -> Anfahrpunkt_5
    Anfahrpunkt_5 -> Wechsel_5 : [abs(x_soll - x_Wagen) <= Zielradius && abs(y_soll - y_Wagen) <= Zielradius]
    Wechsel_5 -> Anfahrpunkt_6
    Anfahrpunkt_6 -> Wechsel_6 : [abs(x_soll - x_Wagen) <= Zielradius && abs(y_soll - y_Wagen) <= Zielradius]
    Wechsel_6 -> Anfahrpunkt_7
    Anfahrpunkt_7 -> Wechsel_7 : [abs(x_soll - x_Wagen) <= Zielradius && abs(y_soll - y_Wagen) <= Zielradius]
    Wechsel_7 -> Anfahrpunkt_8
    Anfahrpunkt_8 -> Wechsel_8 : [abs(x_soll - x_Wagen) <= Zielradius && abs(y_soll - y_Wagen) <= Zielradius]
    Wechsel_8 -> Anfahrpunkt_9
    Anfahrpunkt_9 -> Wechsel_9 : [abs(x_soll - x_Wagen) <= Zielradius && abs(y_soll - y_Wagen) <= Zielradius]
    Wechsel_9 -> Anfahrpunkt_10 [order 2]
    Anfahrpunkt_10 -> Wechsel_10 : [abs(x_soll - x_Wagen) <= Zielradius && abs(y_soll - y_Wagen) <= Zielradius]
    Wechsel_10 -> Anfahrpunkt_11
    Anfahrpunkt_11 -> Wechsel_11 : [abs(x_soll - x_Wagen) <= Zielradius && abs(y_soll - y_Wagen) <= Zielradius]
  state Ende
  (default) -> Start_Einstellung_Init
  Start_Einstellung_Init -> Sammeln : {Gang = 0}
  Sammeln -> Uebergabe : [Counter == 18]
      | {Gang = 1;
      | x_least = x_soll;
      | y_least = y_soll;}
  Uebergabe -> Parken : [Counter == 2]{Gang = 0}
  Parken -> Ende : [Counter == 3]
  data: x_soll output; y_soll output; x_Wagen input; y_Wagen input; Counter local; x_least local; y_least local; Zielradius output; Gang output

== stateflow chart Nexonar_Navigation1/Navigationssystem [Einstellungen moeglich]/Fahrsystem ==
  state Fahren_mit_Ausrichtungsregelung
    entry:
    pwm_out_l = pwm_out - round(pwm_mindern(1) * (pwm_out / 100) ^ 2) * l_mindern;
    pwm_out_r = pwm_out - round(pwm_mindern(1) * (pwm_out / 100) ^ 2) * r_mindern;
    r_l_out_l = 1 - Gang;
    r_l_out_r = 1 - Gang;
  state Start_Warten
  state Drehen_links_max
    entry:
    pwm_out_l = 100;
    pwm_out_r = 100;
    r_l_out_l = 0;
    r_l_out_r = 1;
  state Drehen_rechts_max
    entry:
    pwm_out_l = 100;
    pwm_out_r = 100;
    r_l_out_l = 1;
    r_l_out_r = 0;
  state Drehen_links_gesteuert
    entry:
    pwm_out_l = 59 + abs(alpha_diff_opt);
    pwm_out_r = 59 + abs(alpha_diff_opt);
    r_l_out_l = 0;
    r_l_out_r = 1;
  state Drehen_rechts_gesteuert
    entry:
    pwm_out_l = 59 + abs(alpha_diff_opt);
    pwm_out_r = 59 + abs(alpha_diff_opt);
    r_l_out_l = 1;
    r_l_out_r = 0;
  (junction 81) -> Fahren_mit_Ausrichtungsregelung [order 1] : [pwm_mindern(2) == 1]
      | {l_mindern = 1 - Gang; r_mindern = 0 + Gang;}
  (junction 81) -> Fahren_mit_Ausrichtungsregelung [order 2] : [pwm_mindern(2) == 0]
      | {l_mindern = 0 + Gang; r_mindern = 1 - Gang;}
  (junction 1) -> (junction 81) [order 2]
  Fahren_mit_Ausrichtungsregelung -> (junction 32)
  (junction 81) -> Fahren_mit_Ausrichtungsregelung [order 3] : {l_mindern = 0; r_mindern = 0;}
  Start_Warten -> (junction 1)
  (junction 32) -> (junction 1)
  (default) -> Start_Warten
  Drehen_links_max -> (junction 32)
  Drehen_rechts_max -> (junction 32)
  Drehen_links_gesteuert -> (junction 32)
  (junction 1) -> (junction 18) [order 1] : [abs(alpha_diff_opt) > 0 && pwm_out > 0]
  Drehen_rechts_gesteuert -> (junction 32)
  (junction 18) -> (junction 44) [order 1] : [abs(alpha_diff_opt) > 40]
  (junction 44) -> Drehen_links_max [order 1] : [alpha_diff_opt > 0]
  (junction 18) -> (junction 52) [order 2]
  (junction 44) -> Drehen_rechts_max [order 2]
  (junction 52) -> Drehen_links_gesteuert [order 1] : [alpha_diff_opt > 0]
  (junction 52) -> Drehen_rechts_gesteuert [order 2]
  data: Gang input; pwm_out input; pwm_mindern input; alpha_diff_opt input; pwm_out_l output; pwm_out_r output; r_l_out_l output; r_l_out_r output; l_mindern local; r_mindern local

== stateflow chart Nexonar_Navigation1/Navigationssystem [Einstellungen moeglich]/Drehweg-Optimierung mit Gang-Ausrichtung [Init: Stillstandintervall = ±5°] ==
  state Einstellung_Init
    entry:
    Stillstandintervall = 15;
    %%%
    pwm_mindern = [0 0];
  state Drehstillstand_mit_Ausrichtungsregelung
    entry:
    alpha_diff_opt = 0;
    if abs(alpha_diff_intern) < 5
    pwm_mindern(1) = round(abs(alpha_diff_intern));
    elseif abs(alpha_diff_intern) < 15
    pwm_mindern(1) = 5 + floor((abs(alpha_diff_intern) - 5) / 2);
    else
    pwm_mindern(1) = 10;
    end;
    if alpha_diff_intern < 0
    pwm_mindern(2) = 0;
    elseif alpha_diff_intern > 0
    pwm_mindern(2) = 1;
    else
    pwm_mindern(2) = 2;
    end;
  state Weiterleitung_bei_Drehzustand
    entry:
    alpha_diff_opt = alpha_diff_intern;
  (default) -> Einstellung_Init
  (junction 95) -> (junction 32)
  Einstellung_Init -> (junction 32)
  (junction 32) -> (junction 6) : {alpha_diff_intern = alpha_diff + 180 * Gang}
  (junction 6) -> (junction 68) [order 2]
  (junction 68) -> Drehstillstand_mit_Ausrichtungsregelung [order 1] : [abs(alpha_diff_intern) <= Stillstandintervall]
  Drehstillstand_mit_Ausrichtungsregelung -> (junction 95)
  (junction 6) -> (junction 13) [order 1] : [abs(alpha_diff_intern) > 180]
  (junction 13) -> (junction 68) [order 1] : [alpha_diff_intern > 0]
      | {alpha_diff_intern = -360 + alpha_diff_intern}
  Weiterleitung_bei_Drehzustand -> (junction 95)
  (junction 13) -> (junction 68) [order 2] : {alpha_diff_intern = 360 + alpha_diff_intern}
  (junction 68) -> Weiterleitung_bei_Drehzustand [order 2]
  data: pwm_mindern output; Gang input; alpha_diff input; alpha_diff_opt output; alpha_diff_intern local; Stillstandintervall local

== stateflow chart Nexonar_Navigation1/Navigationssystem [Einstellungen moeglich]/Winkelregelungssystem (Soll-Ist-Abgleich & Ausrichtungsauswertung)/Quadrantenteiler ==
  state Quadrant_a
    entry:
    Quadrant = 0;
  state Quadrant_b
    entry:
    Quadrant = 1;
  state Start_Warten
  state Quadrant_c
    entry:
    Quadrant = 2;
  state Quadrant_d
    entry:
    Quadrant = 3;
  (junction 6) -> Quadrant_a [order 1] : [x_diff >= 0 && y_diff >= 0]
  Quadrant_a -> (junction 35)
  (junction 6) -> Quadrant_b [order 2] : [x_diff <= 0 && y_diff > 0]
  Quadrant_b -> (junction 35)
  Start_Warten -> (junction 6)
  (junction 35) -> (junction 6)
  (default) -> Start_Warten
  (junction 6) -> Quadrant_c [order 3] : [x_diff < 0 && y_diff <= 0]
  Quadrant_c -> (junction 35)
  (junction 6) -> Quadrant_d [order 4]
  Quadrant_d -> (junction 35)
  data: x_diff input; y_diff input; Quadrant output

== stateflow chart Nexonar_Navigation1/Navigationssystem [Einstellungen moeglich]/Winkelregelungssystem (Soll-Ist-Abgleich & Ausrichtungsauswertung)/Winkelausgabe fuer Ausrichtung ==
  state Ausrichtung_ohne_Aenderung
    entry:
    alpha_neu = alpha_Wagen;
  state Start_Warten
  state Trigonometrische_Auswertung_in_Grad_fuer_Quadrant_1_3
    entry:
    alpha_neu = round(atan(abs(x_diff)/abs(y_diff))*360/(2*pi));
  state Trigonometrische_Auswertung_in_Grad_fuer_Quadrant_0_2
    entry:
    alpha_neu = round(atan(abs(y_diff)/abs(x_diff))*360/(2*pi));
  (junction 4) -> Ausrichtung_ohne_Aenderung [order 1] : [x_diff == 0 && y_diff == 0]
  Ausrichtung_ohne_Aenderung -> (junction 65)
  Start_Warten -> (junction 4)
  (junction 65) -> (junction 4)
  (default) -> Start_Warten
  (junction 4) -> Trigonometrische_Auswertung_in_Grad_fuer_Quadrant_1_3 [order 4]
  (junction 4) -> Trigonometrische_Auswertung_in_Grad_fuer_Quadrant_0_2 [order 2] : [x_diff > 0 && y_diff >= 0]
  Trigonometrische_Auswertung_in_Grad_fuer_Quadrant_0_2 -> (junction 65)
  (junction 4) -> Trigonometrische_Auswertung_in_Grad_fuer_Quadrant_0_2 [order 3] : [x_diff < 0 && y_diff <= 0]
  Trigonometrische_Auswertung_in_Grad_fuer_Quadrant_1_3 -> (junction 65)
  data: x_diff input; y_diff input; alpha_neu output; alpha_Wagen input

== stateflow chart Nexonar_Navigation1/Nexonar-Positionsbestimmung/Chart2 ==
  state Daten_einlesen
  state x0
  state x1_1
    entry: int16y_bin[0] = int8y_1[0];
    int16y_bin[1] = int8y_1[1];
    int16y_bin[2] = int8y_1[2];
    int16y_bin[3] = int8y_1[3];
    int16y_bin[4] = int8y_1[4];
    int16y_bin[5] = int8y_1[5]
    int16y_bin[6] = int8y_1[6];
    int16y_bin[7] = int8y_1[7];
    int16y_bin[8] = int8y_2[0];
    int16y_bin[9] = int8y_2[1];
    int16y_bin[10] = int8y_2[2];
    int16y_bin[11] = int8y_2[3];
    int16y_bin[12] = int8y_2[4];
    int16y_bin[13] = int8y_2[5]
    int16y_bin[14] = int8y_2[6];
    int16y_bin[15] = int8y_2[7];
  x0 -> Daten_einlesen
  (default) -> x0
  Daten_einlesen -> x1_1
  x1_1 -> Daten_einlesen
  data: int8y_1 input size=8; int8y_2 input size=8; int16y_bin output size=16 =0

== stateflow chart Nexonar_Navigation1/Nexonar-Positionsbestimmung/Chart4 ==
  state Daten_einlesen
  state x0
  state x1_1
    entry: int16a1_bin[0] = int8a1_1[0];
    int16a1_bin[1] = int8a1_1[1];
    int16a1_bin[2] = int8a1_1[2];
    int16a1_bin[3] = int8a1_1[3];
    int16a1_bin[4] = int8a1_1[4];
    int16a1_bin[5] = int8a1_1[5]
    int16a1_bin[6] = int8a1_1[6];
    int16a1_bin[7] = int8a1_1[7];
    int16a1_bin[8] = int8a1_2[0];
    int16a1_bin[9] = int8a1_2[1];
    int16a1_bin[10] = int8a1_2[2];
    int16a1_bin[11] = int8a1_2[3];
    int16a1_bin[12] = int8a1_2[4];
    int16a1_bin[13] = int8a1_2[5]
    int16a1_bin[14] = int8a1_2[6];
    int16a1_bin[15] = int8a1_2[7];
  x0 -> Daten_einlesen
  (default) -> x0
  Daten_einlesen -> x1_1
  x1_1 -> Daten_einlesen
  data: int8a1_1 input size=8; int8a1_2 input size=8; int16a1_bin output size=16 =0

== stateflow chart Nexonar_Navigation1/Nexonar-Positionsbestimmung/Chart6 ==
  state Daten_einlesen
  state x0
  state x1_1
    entry: int16x_bin[0] = int8x_1[0];
    int16x_bin[1] = int8x_1[1];
    int16x_bin[2] = int8x_1[2];
    int16x_bin[3] = int8x_1[3];
    int16x_bin[4] = int8x_1[4];
    int16x_bin[5] = int8x_1[5]
    int16x_bin[6] = int8x_1[6];
    int16x_bin[7] = int8x_1[7];
    int16x_bin[8] = int8x_2[0];
    int16x_bin[9] = int8x_2[1];
    int16x_bin[10] = int8x_2[2];
    int16x_bin[11] = int8x_2[3];
    int16x_bin[12] = int8x_2[4];
    int16x_bin[13] = int8x_2[5]
    int16x_bin[14] = int8x_2[6];
    int16x_bin[15] = int8x_2[7];
  x0 -> Daten_einlesen
  (default) -> x0
  Daten_einlesen -> x1_1
  x1_1 -> Daten_einlesen
  data: int8x_1 input size=8; int8x_2 input size=8; int16x_bin output size=16 =0

== stateflow chart Nexonar_Navigation1/Nexonar-Positionsbestimmung/Chart8 ==
  state wert_erkannt
    entry:
    values_out1[0] = in_data[0];
    values_out1[1] = in_data[1];
    values_out1[2] = in_data[2];
    values_out1[3] = in_data[3];
    values_out1[4] = in_data[4];
    values_out1[5] = in_data[5];
    values_out1[6] = in_data[6];
    values_out1[7] = in_data[7];
    values_out1[8] = in_data[8];
    values_out1[9] = in_data[9];
    values_out1[10] = in_data[10];
    values_out1[11] = in_data[11];
    values_out1[12] = in_data[12];
    values_out1[13] = in_data[13];
    values_out1[14] = in_data[14];
    values_out1[15] = in_data[15];
    values_out1[16] = in_data[16];
    values_out1[17] = in_data[17];
    values_out1[18] = in_data[18];
    values_out1[19] = in_data[19];
  state init
    entry: values_out1[0] = 0;
    values_out1[1] = 0;
    values_out1[2] = 0;
    values_out1[3] = 0;
    values_out1[4] = 0;
    values_out1[5] = 0;
    values_out1[6] = 0;
    values_out1[7] = 0;
    values_out1[8] = 0;
    values_out1[9] = 0;
    values_out1[10] = 0;
    values_out1[11] = 0;
    values_out1[12] = 0;
    values_out1[13] = 0;
    values_out1[14] = 0;
    values_out1[15] = 0;
    values_out1[16] = 0;
    values_out1[17] = 0;
    values_out1[18] = 0;
    values_out1[19] = 0;
  state Anfang_found_Schritt_uebertragen_weglassen_performance
    entry: x_found = x_found +1;
  state x5_valid_data_found1
    entry: valid_values1 = values_out1[search+1];
    valid_values2 = values_out1[search+2];
    valid_values3 = values_out1[search+3];
    valid_values4 = values_out1[search+4];
    valid_values5 = values_out1[search+5];
    valid_values6 = values_out1[search+6];
    valid_values7 = values_out1[search+7];
    valid_values8 = values_out1[search+8];
    zaehler = zaehler +1;
  state wert_erkannt2
    entry:
    search = 0;
    counter = counter + 1;
  state x1_search1
    entry: search = search + 1;
  x5_valid_data_found1 -> wert_erkannt
  (default) -> init
  x1_search1 -> wert_erkannt [order 3]
  init -> wert_erkannt
  Anfang_found_Schritt_uebertragen_weglassen_performance -> x5_valid_data_found1 [order 1] : [((values_out1[search]+values_out1[search+1]+values_out1[search+2]+values_out1[search+3]+values_out1[search+4]+values_out1[search+5]+values_out1[search+6]+values_out1[search+7]+values_out1[search+8])) == values_out1[search+9]]
  Anfang_found_Schritt_uebertragen_weglassen_performance -> x5_valid_data_found1 [order 2] : [((values_out1[search]+values_out1[search+1]+values_out1[search+2]+values_out1[search+3]+values_out1[search+4]+values_out1[search+5]+values_out1[search+6]+values_out1[search+7]+values_out1[search+8])-(256)) == values_out1[search+9]]
  wert_erkannt -> wert_erkannt2
  Anfang_found_Schritt_uebertragen_weglassen_performance -> x5_valid_data_found1 [order 3] : [((values_out1[search]+values_out1[search+1]+values_out1[search+2]+values_out1[search+3]+values_out1[search+4]+values_out1[search+5]+values_out1[search+6]+values_out1[search+7]+values_out1[search+8])-(512)) == values_out1[search+9]]
  Anfang_found_Schritt_uebertragen_weglassen_performance -> x5_valid_data_found1 [order 7] : [((values_out1[search]+values_out1[search+1]+values_out1[search+2]+values_out1[search+3]+values_out1[search+4]+values_out1[search+5]+values_out1[search+6]+values_out1[search+7]+values_out1[search+8])-(768)) == values_out1[search+9]]
  Anfang_found_Schritt_uebertragen_weglassen_performance -> x5_valid_data_found1 [order 6] : [((values_out1[search]+values_out1[search+1]+values_out1[search+2]+values_out1[search+3]+values_out1[search+4]+values_out1[search+5]+values_out1[search+6]+values_out1[search+7]+values_out1[search+8])-(1024)) == values_out1[search+9]]
  Anfang_found_Schritt_uebertragen_weglassen_performance -> x5_valid_data_found1 [order 5] : [((values_out1[search]+values_out1[search+1]+values_out1[search+2]+values_out1[search+3]+values_out1[search+4]+values_out1[search+5]+values_out1[search+6]+values_out1[search+7]+values_out1[search+8])-(1280)) == values_out1[search+9]]
  Anfang_found_Schritt_uebertragen_weglassen_performance -> x5_valid_data_found1 [order 4] : [((values_out1[search]+values_out1[search+1]+values_out1[search+2]+values_out1[search+3]+values_out1[search+4]+values_out1[search+5]+values_out1[search+6]+values_out1[search+7]+values_out1[search+8])-(1536)) == values_out1[search+9]]
  Anfang_found_Schritt_uebertragen_weglassen_performance -> x5_valid_data_found1 [order 8] : [((values_out1[search]+values_out1[search+1]+values_out1[search+2]+values_out1[search+3]+values_out1[search+4]+values_out1[search+5]+values_out1[search+6]+values_out1[search+7]+values_out1[search+8])-(1792)) == values_out1[search+9]]
  Anfang_found_Schritt_uebertragen_weglassen_performance -> x5_valid_data_found1 [order 10] : [((values_out1[search]+values_out1[search+1]+values_out1[search+2]+values_out1[search+3]+values_out1[search+4]+values_out1[search+5]+values_out1[search+6]+values_out1[search+7]+values_out1[search+8])-(2048)) == values_out1[search+9]]
  Anfang_found_Schritt_uebertragen_weglassen_performance -> x1_search1 [order 9]
  wert_erkannt2 -> Anfang_found_Schritt_uebertragen_weglassen_performance [order 1] : [values_out1[search] == 88]
  x1_search1 -> Anfang_found_Schritt_uebertragen_weglassen_performance [order 1] : [values_out1[search] == 88]
  wert_erkannt2 -> x1_search1 [order 2]
  x1_search1 -> x1_search1 [order 2] : [search < 19]
  data: in_data input size=20; values_out1 local int16 size=20; zaehler local int32 =0; search local int16; valid_values1 output int16 size=1; valid_values2 output int16 size=1; valid_values3 output int16 size=1; valid_values4 output int16 size=1; valid_values5 output int16 size=1; valid_values6 output int16 size=1; valid_values7 output int16 size=1; valid_values8 output int16 size=1; counter local int32 =0; x_found local int32 =0

== matlab function Nexonar_Navigation1/Navigationssystem [Einstellungen moeglich]/Positionsregelungssystem (Soll-Ist-Abgleich & PWM-Auswertung)/Betrag pwm_x ==
  settings: updateMethod=DISCRETE  sampleTime=0.01
  data: x_diff_abs input; pwm_x output; Zielradius input
function pwm_x = fcn( x_diff_abs, Zielradius)

if Zielradius < x_diff_abs && x_diff_abs < 60 + Zielradius
    pwm_x = 60;
elseif x_diff_abs <= Zielradius
    pwm_x = 0;
elseif x_diff_abs >= 100 + Zielradius
    pwm_x = 100;
else
    pwm_x = x_diff_abs;
end

== matlab function Nexonar_Navigation1/Navigationssystem [Einstellungen moeglich]/Positionsregelungssystem (Soll-Ist-Abgleich & PWM-Auswertung)/Betrag pwm_y ==
  settings: updateMethod=DISCRETE  sampleTime=0.01
  data: Zielradius input; y_diff_abs input; pwm_y output
function pwm_y = fcn(Zielradius, y_diff_abs)

if Zielradius < y_diff_abs && y_diff_abs < 60 + Zielradius
    pwm_y = 60;
elseif y_diff_abs <= Zielradius
    pwm_y = 0;
elseif y_diff_abs >= 100 + Zielradius
    pwm_y = 100;
else
    pwm_y = y_diff_abs;
end

== matlab function Nexonar_Navigation1/Nexonar-Positionsbestimmung/I2C Reset (behebt Stabilitätsprobleme der I2C-Verbindung)/I2C Reset/I2C Reset ==
function fcn()
%#codegen

coder.ceval( 'reset_i2c' );

== matlab function Nexonar_Navigation1/Nexonar-Positionsbestimmung/I2C Reset (behebt Stabilitätsprobleme der I2C-Verbindung)/I2C Reinitialisierung/I2C Reinitialisierung ==
function fcn()
%#codegen

coder.ceval( 'init_i2c' );
